simulink model "and_or_combinational_dashboard"  (R2018b)
settings: Solver=VariableStepAuto  StartTime=0.0  StopTime=30  RelTol=1e-3
settings Model: EnablePacing=on  Creator=kjartan  LastModifiedBy=kjartan

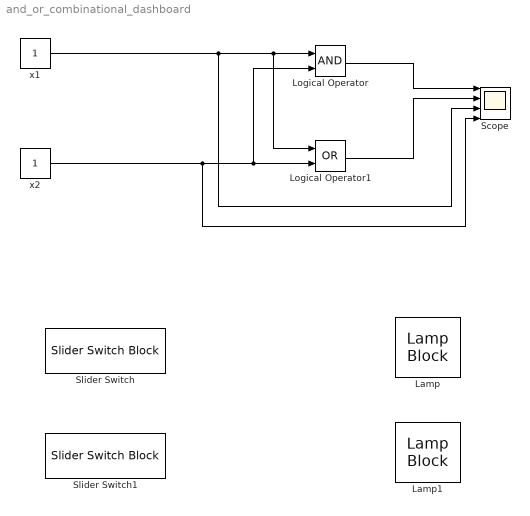
== system and_or_combinational_dashboard ==
  Lamp : LampBlock  WebBlockId=9
  Lamp1 : LampBlock  WebBlockId=10
  Logical Operator : Logic  AllPortsSameDT=off  OutDataTypeStr=boolean
  Logical Operator1 : Logic  Operator=OR  AllPortsSameDT=off  OutDataTypeStr=boolean
  Scope : Scope  NumInputPorts=4
  Slider Switch : SliderSwitchBlock  WebBlockId=12
      settings: Values={{'Off', 'On'}, [0 1]}
  Slider Switch1 : SliderSwitchBlock  WebBlockId=13
      settings: Values={{'Off', 'On'}, [0 1]}
  x1 : Constant
  x2 : Constant
  wires:
  x1/1 -> Scope/3, Logical Operator1/1, Logical Operator/1
  x2/1 -> Scope/4, Logical Operator1/2, Logical Operator/2
  Logical Operator/1 -> Scope/1
  Logical Operator1/1 -> Scope/2
